simulink model "mechanical_reduced_order_to_pdf"  (R2015b)
settings: Solver=VariableStepAuto  StartTime=0.0  StopTime=10.0  RelTol=1e-3
undefined symbols (not defined in the file): L, R, Vin
settings Model: Creator=Morten  LastModifiedBy=Morten

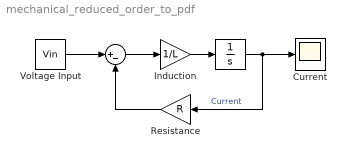
== system mechanical_reduced_order_to_pdf ==
  "     " : Sum  Inputs=|+-
  "               " : Integrator
  Current : Scope
  "Induction  " : Gain  Gain=1/L
  "Resistance  " : Gain  Gain=R
  Voltage Input : Constant  Value=Vin
  wires:
  "     "/1 -> "Induction  "/1
  "Resistance  "/1 -> "     "/2
  "               "/1 -> Current/1, "Resistance  "/1  "Current"
  "Induction  "/1 -> "               "/1
  Voltage Input/1 -> "     "/1
